simulink model "modelo_mpc_com_restricao_estimador"  (R2018b)
settings: Solver=VariableStepAuto  StartTime=0.0  StopTime=50  RelTol=1e-3
values from neighbouring files (symbols this model uses):
  A = [0 1 0 0 ... (first row only)    [dadosBallBeam.m]    (also in dadosTanqueQuatro.m = [-1/T1 0 A3/(A1*T3) 0; tanqueQuatroLinearizacao.m = double(subs(As,{h1,h2,h3,h4,v1,v2},{h10,h20,h30,h40,v10,v20})
  A1 = 28    [dadosTanqueQuatro.m]    (also in tanqueQuatroLinearizacao.m)
  a1 = 0.071    [dadosTanqueQuatro.m]    (also in tanqueQuatroLinearizacao.m)
  A2 = 32    [dadosTanqueQuatro.m]    (also in tanqueQuatroLinearizacao.m)
  a2 = 0.057    [dadosTanqueQuatro.m]    (also in tanqueQuatroLinearizacao.m)
  a3 = 0.071    [dadosTanqueQuatro.m]    (also in tanqueQuatroLinearizacao.m)
  A3 = 28    [dadosTanqueQuatro.m]    (also in tanqueQuatroLinearizacao.m)
  a4 = 0.057    [dadosTanqueQuatro.m]    (also in tanqueQuatroLinearizacao.m)
  A4 = 32    [dadosTanqueQuatro.m]    (also in tanqueQuatroLinearizacao.m)
  Aa = [Ad, zeros(m,n_saidas); Cd*Ad, eye(n_saidas)]    [MPC_sem_restricao.m]    (also in dados_MPC_com_restricao.m; dados_MPC_com_restricao_estimador.m; dados_MPC_sem_restricao.m; dados_MPC_sem_restricao_estimador.m)
  B = [0 0 0 1]'    [dadosBallBeam.m]    (also in dadosTanqueQuatro.m = [(y1*k1)/A1 0; tanqueQuatroLinearizacao.m = double(subs(Bs,{h1,h2,h3,h4,v1,v2},{h10,h20,h30,h40,v10,v20})
  Ba = [Bd;Cd*Bd]    [MPC_sem_restricao.m]    (also in dados_MPC_com_restricao.m; dados_MPC_com_restricao_estimador.m; dados_MPC_sem_restricao.m; dados_MPC_sem_restricao_estimador.m)
  C = [1 0 0 0]    [dadosBallBeam.m]    (also in dadosTanqueQuatro.m = [1 0 0 0; tanqueQuatroLinearizacao.m = [1 0 0 0)
  D = [0]    [dadosBallBeam.m]    (also in dadosTanqueQuatro.m = [0 0; tanqueQuatroLinearizacao.m = [0 0)
  g = -9.8    [dadosBallBeam.m]    (also in dadosTanqueQuatro.m = 981; tanqueQuatroLinearizacao.m = 981)
  h1 = 12.4    [dadosTanqueQuatro.m]
  h2 = 12.7    [dadosTanqueQuatro.m]
  h3 = 1.8    [dadosTanqueQuatro.m]
  h4 = 1.4    [dadosTanqueQuatro.m]
  Ha = [H zeros(n_saidas,size(H,1)); zeros(n_saidas,size(H,2)) eye(n_saidas)]    [dados_MPC_com_restricao_estimador.m]    (also in dados_MPC_sem_restricao_estimador.m)
  k1 = 3.33    [dadosTanqueQuatro.m]    (also in tanqueQuatroLinearizacao.m)
  k2 = 3.35    [dadosTanqueQuatro.m]    (also in tanqueQuatroLinearizacao.m)
  L = 1.0    (= 1)    [dadosBallBeam.m]    (also in dados_MPC_com_restricao_estimador.m = Lt'; dados_MPC_sem_restricao_estimador.m = Lt')
  ts = 0.1    [dados_MPC_com_restricao.m]    (also in dados_MPC_com_restricao_estimador.m; dados_MPC_sem_restricao.m; dados_MPC_sem_restricao_estimador.m)
  v1 = 3    [dadosTanqueQuatro.m]
  v2 = 3    [dadosTanqueQuatro.m]
  y1 = 0.7    [dadosTanqueQuatro.m]
  y2 = 0.6    [dadosTanqueQuatro.m]
undefined symbols (not defined in the file or in its folder): DiscIntNeverNeededParam, var
libraries: simulink x2
settings Model: Creator=Caléo  LastModifiedBy=Caléo

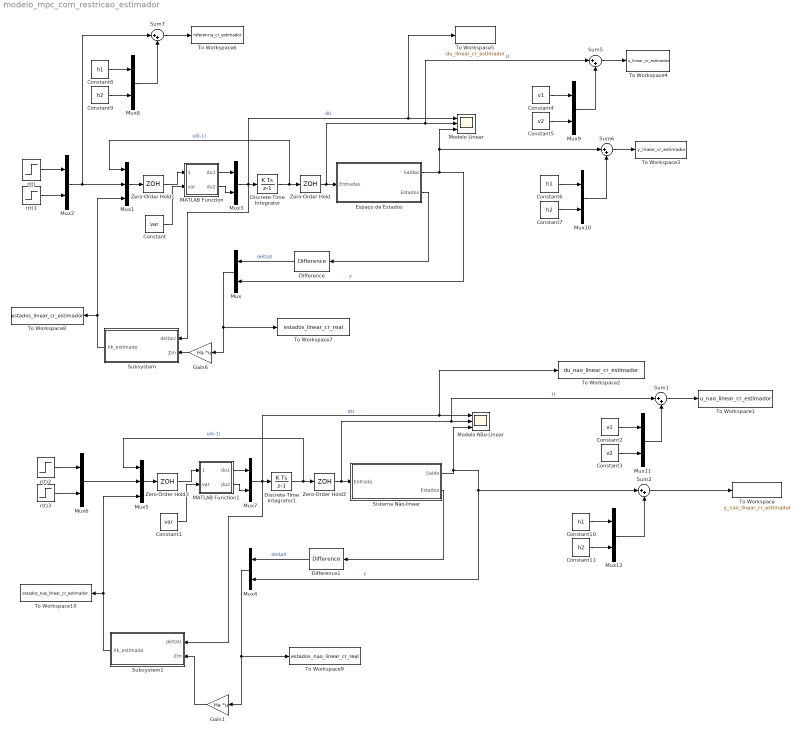
== system modelo_mpc_com_restricao_estimador ==
  Constant : Constant  Value=var  OutDataTypeStr=Bus: var_bus
  Constant1 : Constant  Value=var  OutDataTypeStr=Bus: var_bus
  Constant10 : Constant  Value=h1
  Constant11 : Constant  Value=h2
  Constant2 : Constant  Value=v1
  Constant3 : Constant  Value=v2
  Constant4 : Constant  Value=v1
  Constant5 : Constant  Value=v2
  Constant6 : Constant  Value=h1
  Constant7 : Constant  Value=h2
  Constant8 : Constant  Value=h1
  Constant9 : Constant  Value=h2
  Difference : simulink/Discrete/Difference  ICPrevInput=0.0  OutMin=[]  OutMax=[]  OutDataType=fixdt(1, 16)  OutScaling=2^-10  DoSatur=off
  Difference1 : simulink/Discrete/Difference  ICPrevInput=0.0  OutMin=[]  OutMax=[]  OutDataType=fixdt(1, 16)  OutScaling=2^-10  DoSatur=off
  Discrete-Time Integrator : DiscreteIntegrator  SampleTime=ts  ICPrevOutput=DiscIntNeverNeededParam  ICPrevScaledInput=DiscIntNeverNeededParam
  Discrete-Time Integrator1 : DiscreteIntegrator  SampleTime=ts  ICPrevOutput=DiscIntNeverNeededParam  ICPrevScaledInput=DiscIntNeverNeededParam
  Espaço de Estados : Subsystem
  Gain1 : Gain  Gain=Ha  Multiplication=Matrix(K*u)
  Gain6 : Gain  Gain=Ha  Multiplication=Matrix(K*u)
  MATLAB Function : MATLAB Function  TreatAsAtomicUnit=on
  MATLAB Function1 : MATLAB Function  TreatAsAtomicUnit=on
  Modelo Linear : Scope  NumInputPorts=3
  Modelo Não-Linear : Scope  NumInputPorts=3
  Mux{,2..4,6..12} (11 alike) : Mux  Inputs=2
  Mux1 : Mux  Inputs=3
  Mux5 : Mux  Inputs=3
  Sistema Não-linear : Subsystem
  Subsystem : Subsystem
  Subsystem1 : Subsystem
  Sum{1..2,5..7} (5 alike) : Sum  Inputs=|++
  To Workspace : ToWorkspace  VariableName=y_nao_linear_cr_estimador  SaveFormat=Timeseries  SampleTime=-1
  To Workspace1 : ToWorkspace  VariableName=u_nao_linear_cr_estimador  SaveFormat=Timeseries  SampleTime=-1
  To Workspace10 : ToWorkspace  VariableName=estados_nao_linear_cr_estimador  SaveFormat=Timeseries  SampleTime=-1
  To Workspace2 : ToWorkspace  VariableName=du_nao_linear_cr_estimador  SaveFormat=Timeseries  SampleTime=-1
  To Workspace3 : ToWorkspace  VariableName=y_linear_cr_estimador  SaveFormat=Timeseries  SampleTime=-1
  To Workspace4 : ToWorkspace  VariableName=u_linear_cr_estimador  SaveFormat=Timeseries  SampleTime=-1
  To Workspace5 : ToWorkspace  VariableName=du_linear_cr_estimador  SaveFormat=Timeseries  SampleTime=-1
  To Workspace6 : ToWorkspace  VariableName=referencia_cr_estimador  SaveFormat=Timeseries  SampleTime=-1
  To Workspace7 : ToWorkspace  VariableName=estados_linear_cr_real  SaveFormat=Timeseries  SampleTime=-1
  To Workspace8 : ToWorkspace  VariableName=estados_linear_cr_estimador  SaveFormat=Timeseries  SampleTime=-1
  To Workspace9 : ToWorkspace  VariableName=estados_nao_linear_cr_real  SaveFormat=Timeseries  SampleTime=-1
  Zero-Order Hold{,1..3} (4 alike) : ZeroOrderHold  SampleTime=ts
  r(t) : Step  Time=0  After=2  SampleTime=0
  r(t)1 : Step  Time=0  After=-0.5  SampleTime=0
  r(t)2 : Step  Time=0  After=2  SampleTime=0
  r(t)3 : Step  Time=0  After=-0.5  SampleTime=0
  wires:
  Espaço de Estados/1(Saídas) -> Sum6/1, Modelo Linear/3, Mux/2  "Y"
  Difference/1 -> Mux/1  "deltaX"
  Espaço de Estados/2(Estados) -> Difference/1
  Discrete-Time Integrator/1 -> Mux1/1, Zero-Order Hold/1  "u(k-1)"
  r(t)/1 -> Mux2/1
  r(t)1/1 -> Mux2/2
  Mux1/1 -> Zero-Order Hold1/1
  Zero-Order Hold1/1 -> MATLAB Function/1(entrada)
  Constant/1 -> MATLAB Function/2(var)
  MATLAB Function/1(du1) -> Mux3/1
  MATLAB Function/2(du2) -> Mux3/2
  MATLAB Function1/1(du1) -> Mux7/1
  r(t)3/1 -> Mux6/2
  r(t)2/1 -> Mux6/1
  Zero-Order Hold2/1 -> Sistema Não-linear/1(Entrada), Sum1/1, Modelo Não-Linear/2  "U"
  Constant1/1 -> MATLAB Function1/2(var)
  MATLAB Function1/2(du2) -> Mux7/2
  Mux6/1 -> Mux5/2
  Discrete-Time Integrator1/1 -> Mux5/1, Zero-Order Hold2/1  "u(k-1)"
  Sistema Não-linear/1("Saída ") -> Modelo Não-Linear/3, Mux4/2, Sum2/1  "Y"
  Mux5/1 -> Zero-Order Hold3/1
  Zero-Order Hold3/1 -> MATLAB Function1/1(entrada)
  Sistema Não-linear/2("Estados ") -> Difference1/1
  Difference1/1 -> Mux4/1  "deltaX"
  Mux3/1 -> Subsystem/1(deltaU), To Workspace5/1, Modelo Linear/1, Discrete-Time Integrator/1  "dU"
  Zero-Order Hold/1 -> Sum5/1, Modelo Linear/2, Espaço de Estados/1(Entradas)  "U"
  Mux2/1 -> Sum7/1, Mux1/2
  Mux8/1 -> Sum7/2
  Constant9/1 -> Mux8/2
  Sum7/1 -> To Workspace6/1
  Constant8/1 -> Mux8/1
  Mux9/1 -> Sum5/2
  Constant4/1 -> Mux9/1
  Constant5/1 -> Mux9/2
  Sum5/1 -> To Workspace4/1
  Constant6/1 -> Mux10/1
  Mux10/1 -> Sum6/2
  Constant7/1 -> Mux10/2
  Sum6/1 -> To Workspace3/1
  Mux11/1 -> Sum1/2
  Constant2/1 -> Mux11/1
  Constant3/1 -> Mux11/2
  Sum1/1 -> To Workspace1/1
  Constant10/1 -> Mux12/1
  Mux12/1 -> Sum2/2
  Constant11/1 -> Mux12/2
  Sum2/1 -> To Workspace/1
  Gain6/1 -> Subsystem/2(Zm)
  Subsystem/1(Xk_estimado) -> To Workspace8/1, Mux1/3
  Mux/1 -> To Workspace7/1, Gain6/1
  Mux7/1 -> Subsystem1/1(deltaU), To Workspace2/1, Modelo Não-Linear/1, Discrete-Time Integrator1/1  "dU"
  Mux4/1 -> To Workspace9/1, Gain1/1
  Subsystem1/1(Xk_estimado) -> To Workspace10/1, Mux5/3
  Gain1/1 -> Subsystem1/2(Zm)

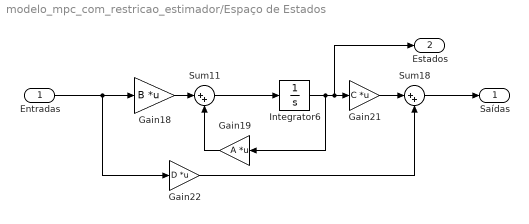
== system modelo_mpc_com_restricao_estimador/Espaço de Estados ==
  Entradas : Inport
  Gain18 : Gain  Gain=B  Multiplication=Matrix(K*u)
  Gain19 : Gain  Gain=A  Multiplication=Matrix(K*u)
  Gain21 : Gain  Gain=C  Multiplication=Matrix(K*u)
  Gain22 : Gain  Gain=D  Multiplication=Matrix(K*u)
  Integrator6 : Integrator
  Sum11 : Sum  Inputs=|++
  Sum18 : Sum  Inputs=|++
  Saídas : Outport
  Estados : Outport  Port=2
  wires:
  Entradas/1 -> Gain22/1, Gain18/1
  Sum18/1 -> Saídas/1
  Gain22/1 -> Sum18/2
  Gain18/1 -> Sum11/1
  Gain19/1 -> Sum11/2
  Integrator6/1 -> Gain19/1, Estados/1, Gain21/1
  Sum11/1 -> Integrator6/1
  Gain21/1 -> Sum18/1

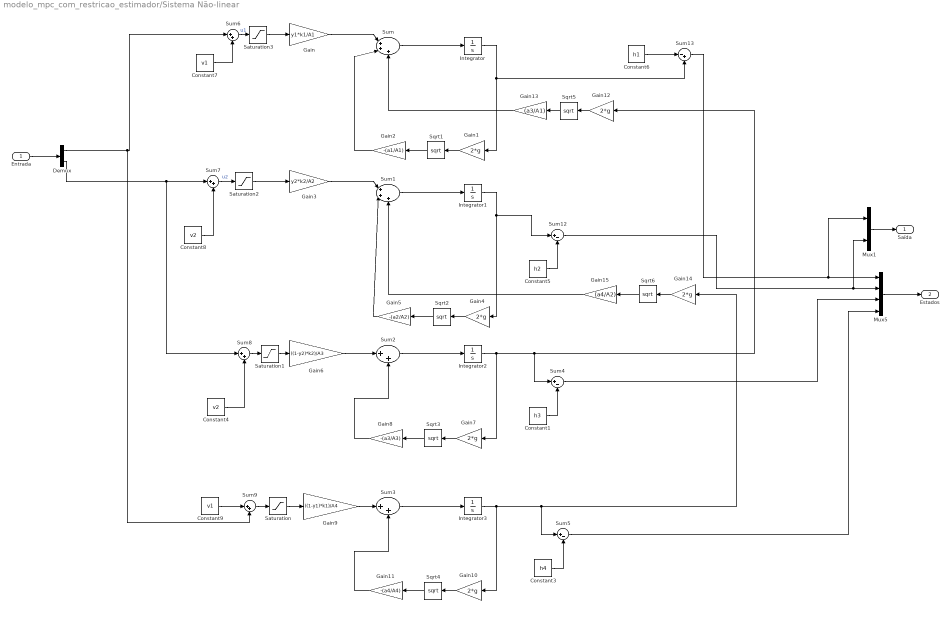
== system modelo_mpc_com_restricao_estimador/Sistema Não-linear ==
  Entrada : Inport
  Constant1 : Constant  Value=h3
  Constant3 : Constant  Value=h4
  Constant4 : Constant  Value=v2
  Constant5 : Constant  Value=h2
  Constant6 : Constant  Value=h1
  Constant7 : Constant  Value=v1
  Constant8 : Constant  Value=v2
  Constant9 : Constant  Value=v1
  Demux : Demux  Outputs=2
  Gain : Gain  Gain=y1*k1/A1
  Gain{1,4,7,10,12,14} (6 alike) : Gain  Gain=2*g
  Gain11 : Gain  Gain=-(a4/A4)
  Gain13 : Gain  Gain=(a3/A1)
  Gain15 : Gain  Gain=(a4/A2)
  Gain2 : Gain  Gain=-(a1/A1)
  Gain3 : Gain  Gain=y2*k2/A2
  Gain5 : Gain  Gain=-(a2/A2)
  Gain6 : Gain  Gain=((1-y2)*k2)/A3
  Gain8 : Gain  Gain=-(a3/A3)
  Gain9 : Gain  Gain=((1-y1)*k1)/A4
  Integrator : Integrator  InitialCondition=h1  LimitOutput=on  UpperSaturationLimit=20  LowerSaturationLimit=0
  Integrator1 : Integrator  InitialCondition=h2  LimitOutput=on  UpperSaturationLimit=20  LowerSaturationLimit=0
  Integrator2 : Integrator  InitialCondition=h3  LimitOutput=on  UpperSaturationLimit=20  LowerSaturationLimit=0
  Integrator3 : Integrator  InitialCondition=h4  LimitOutput=on  UpperSaturationLimit=20  LowerSaturationLimit=0
  Mux1 : Mux  Inputs=2
  Mux5 : Mux
  Saturation{,1..3} (4 alike) : Saturate  UpperLimit=12  LowerLimit=0
  Sqrt{1..6} (6 alike) : Sqrt  SaturateOnIntegerOverflow=on
  Sum : Sum  Inputs=|+++
  Sum1 : Sum  Inputs=|+++
  Sum12 : Sum  Inputs=|+-
  Sum13 : Sum  Inputs=|-+
  Sum{2..3,6..9} (6 alike) : Sum  Inputs=|++
  Sum4 : Sum  Inputs=|+-
  Sum5 : Sum  Inputs=|+-
  "Saída " : Outport
  "Estados " : Outport  Port=2
  wires:
  Demux/1 -> Sum9/2, Sum6/1
  Demux/2 -> Sum8/1, Sum7/1
  Mux1/1 -> "Saída "/1
  Constant9/1 -> Sum9/1
  Sum8/1 -> Saturation1/1
  Entrada/1 -> Demux/1
  Sum5/1 -> Mux5/4
  Sum13/1 -> Mux1/1, Mux5/1
  Gain8/1 -> Sum2/2
  Sqrt5/1 -> Gain13/1
  Gain12/1 -> Sqrt5/1
  Integrator3/1 -> Sum5/1, Gain14/1, Gain10/1
  Saturation3/1 -> Gain/1
  Sqrt2/1 -> Gain5/1
  Integrator2/1 -> Sum4/1, Gain12/1, Gain7/1
  Constant6/1 -> Sum13/1
  Sum4/1 -> Mux5/3
  Sqrt1/1 -> Gain2/1
  Gain9/1 -> Sum3/1
  Gain14/1 -> Sqrt6/1
  Sum3/1 -> Integrator3/1
  Gain/1 -> Sum/1
  Gain7/1 -> Sqrt3/1
  Gain13/1 -> Sum/3
  Constant8/1 -> Sum7/2
  Integrator/1 -> Sum13/2, Gain1/1
  Gain6/1 -> Sum2/1
  Saturation1/1 -> Gain6/1
  Saturation/1 -> Gain9/1
  Sqrt6/1 -> Gain15/1
  Constant1/1 -> Sum4/2
  Constant7/1 -> Sum6/2
  Integrator1/1 -> Gain4/1, Sum12/1
  Sqrt4/1 -> Gain11/1
  Sum6/1 -> Saturation3/1  "u1"
  Sqrt3/1 -> Gain8/1
  Gain2/1 -> Sum/2
  Sum2/1 -> Integrator2/1
  Gain5/1 -> Sum1/2
  Gain3/1 -> Sum1/1
  Sum7/1 -> Saturation2/1  "u2"
  Gain1/1 -> Sqrt1/1
  Mux5/1 -> "Estados "/1
  Sum1/1 -> Integrator1/1
  Sum12/1 -> Mux1/2, Mux5/2
  Gain4/1 -> Sqrt2/1
  Gain11/1 -> Sum3/2
  Sum/1 -> Integrator/1
  Constant5/1 -> Sum12/2
  Gain15/1 -> Sum1/3
  Gain10/1 -> Sqrt4/1
  Constant4/1 -> Sum8/2
  Constant3/1 -> Sum5/2
  Sum9/1 -> Saturation/1
  Saturation2/1 -> Gain3/1

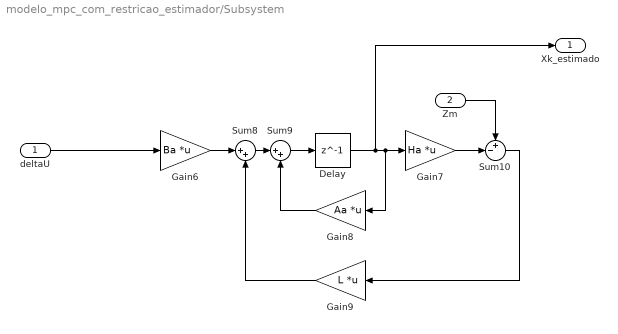
== system modelo_mpc_com_restricao_estimador/Subsystem ==
  deltaU : Inport
  Zm : Inport  Port=2
  Delay : Delay  DelayLength=1  InitialCondition=0
  Gain6 : Gain  Gain=Ba  Multiplication=Matrix(K*u)
  Gain7 : Gain  Gain=Ha  Multiplication=Matrix(K*u)
  Gain8 : Gain  Gain=Aa  Multiplication=Matrix(K*u)
  Gain9 : Gain  Gain=L  Multiplication=Matrix(K*u)
  Sum10 : Sum  Inputs=+-|
  Sum8 : Sum  Inputs=|++
  Sum9 : Sum  Inputs=|++
  Xk_estimado : Outport
  wires:
  Gain6/1 -> Sum8/1
  Delay/1 -> Xk_estimado/1, Gain8/1, Gain7/1
  Gain7/1 -> Sum10/2
  Sum9/1 -> Delay/1
  Gain8/1 -> Sum9/2
  Sum8/1 -> Sum9/1
  deltaU/1 -> Gain6/1
  Sum10/1 -> Gain9/1
  Zm/1 -> Sum10/1
  Gain9/1 -> Sum8/2

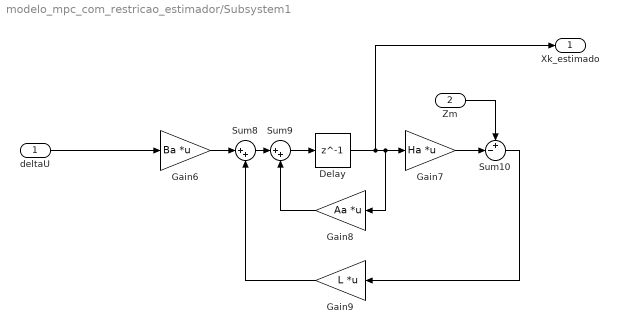
== system modelo_mpc_com_restricao_estimador/Subsystem1 ==
  deltaU : Inport
  Zm : Inport  Port=2
  Delay : Delay  DelayLength=1  InitialCondition=0
  Gain6 : Gain  Gain=Ba  Multiplication=Matrix(K*u)
  Gain7 : Gain  Gain=Ha  Multiplication=Matrix(K*u)
  Gain8 : Gain  Gain=Aa  Multiplication=Matrix(K*u)
  Gain9 : Gain  Gain=L  Multiplication=Matrix(K*u)
  Sum10 : Sum  Inputs=+-|
  Sum8 : Sum  Inputs=|++
  Sum9 : Sum  Inputs=|++
  Xk_estimado : Outport
  wires:
  Gain6/1 -> Sum8/1
  Delay/1 -> Xk_estimado/1, Gain8/1, Gain7/1
  Gain7/1 -> Sum10/2
  Sum9/1 -> Delay/1
  Gain8/1 -> Sum9/2
  Sum8/1 -> Sum9/1
  deltaU/1 -> Gain6/1
  Sum10/1 -> Gain9/1
  Zm/1 -> Sum10/1
  Gain9/1 -> Sum8/2

== matlab function modelo_mpc_com_restricao_estimador/MATLAB Function1 ==
  data: entrada input; du1 output; du2 output; var input
function [du1,du2]  = MPC_com_restricao(entrada,var)
%#codegen
du1 = 0;
du2 = 0;

coder.extrinsic('quadprog');
[N,Nu,Bp,Cp,Qp,Rp,Ap,Ya,Yb,Ua,Ub,M,Dua,Dub] = deal(var.N,var.Nu,var.Bp,var.Cp,var.Qp,var.Rp,var.Ap,var.Ya,var.Yb,var.Ua,var.Ub,var.M,var.Dua,var.Dub);

up = entrada(1:2);
w = entrada(3:4);
Xk = entrada(5:end);


W = repmat(w,N,1);
H = 2*(Bp'*Cp'*Qp*Cp*Bp + Rp);
f = 2*(Qp*Cp*Bp)'*(Cp*Ap*Xk - W);

Um = repmat(up,Nu,1);


Ra = [Ya*Cp*Bp;Ua*M;Dua];
Rb = [Yb-Ya*Cp*Ap*Xk;Ub-Ua*Um;Dub];
% Ra = [Ya*Cp*Bp;Dua];
% Rb = [Yb-Ya*Cp*Ap*Xk;Dub];
du = quadprog(H,f,Ra,Rb);

du1 = du(1);
du2 = du(2);
end

== matlab function modelo_mpc_com_restricao_estimador/MATLAB Function ==
  data: entrada input; du1 output; du2 output; var input
function [du1,du2]  = MPC_com_restricao(entrada,var)
%#codegen
du1 = 0;
du2 = 0;

coder.extrinsic('quadprog');
[N,Nu,Bp,Cp,Qp,Rp,Ap,Ya,Yb,Ua,Ub,M,Dua,Dub] = deal(var.N,var.Nu,var.Bp,var.Cp,var.Qp,var.Rp,var.Ap,var.Ya,var.Yb,var.Ua,var.Ub,var.M,var.Dua,var.Dub);

up = entrada(1:2);
w = entrada(3:4);
Xk = entrada(5:end);


W = repmat(w,N,1);
H = 2*(Bp'*Cp'*Qp*Cp*Bp + Rp);
f = 2*(Qp*Cp*Bp)'*(Cp*Ap*Xk - W);

Um = repmat(up,Nu,1);


Ra = [Ya*Cp*Bp;Ua*M;Dua];
Rb = [Yb-Ya*Cp*Ap*Xk;Ub-Ua*Um;Dub];
% Ra = [Ya*Cp*Bp;Dua];
% Rb = [Yb-Ya*Cp*Ap*Xk;Dub];
du = quadprog(H,f,Ra,Rb);

du1 = du(1);
du2 = du(2);
end
